simulink model "SchematD"  (Simulink 9.2)
settings: Solver=VariableStepAuto  StartTime=0.0  StopTime=10.0  RelTol=1e-3
libraries: simulink_extras x2
settings Model: Creator=bartl  LastModifiedBy=bartl
settings DataIOCC: LimitDataPoints=off  SaveFormat=Dataset  SignalLoggingSaveFormat=Dataset
settings OptimizationCC: LifeSpan=auto
settings DebuggingCC: UnderspecifiedInitializationDetection=Simplified  MergeDetectMultiDrivingBlocksExec=error  FcnCallInpInsideContextMsg=error  StateNameClashWarn=none  SFUnexpectedBacktrackingDiag=error  SFNoUnconditionalDefaultTransitionDiag=error  SFExecutionAtInitializationDiag=warning
settings HardwareCC: ProdBitPerPointer=64  ProdBitPerSizeT=64  ProdBitPerPtrDiffT=64  ProdLargestAtomicFloat=Float  ProdIntDivRoundTo=Zero  ProdEndianess=LittleEndian  ProdWordSize=64  ProdHWDeviceType=Intel->x86-64 (Windows64)
settings ModelReferenceCC: PropagateSignalLabelsOutOfModel=on
settings SFSimCC: SimUseLocalCustomCode=on
settings RTWCC: RTWUseLocalCustomCode=on
settings CodeAppCC: StateflowObjectComments=off
settings GRTTargetCC: TargetLangStandard=C99 (ISO)  GeneratePreprocessorConditionals=Use local settings  CombineOutputUpdateFcns=on  GRTInterface=off
settings ConfigComp: CovMetricSettings=dwe  CovHtmlReporting=off  CovSaveCumulativeToWorkspaceVar=off  CovSaveSingleToWorkspaceVar=off  CovExternalEMLEnable=on

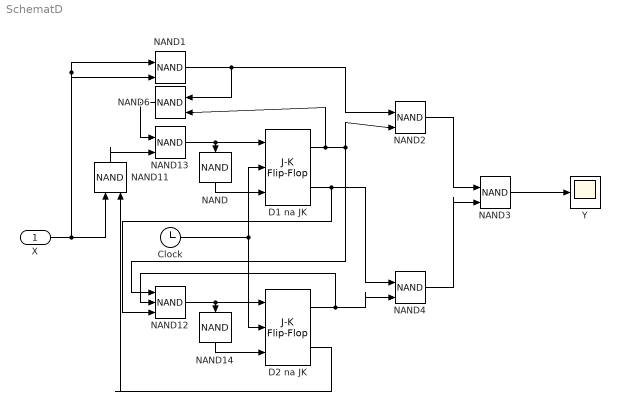
== system SchematD ==
  X : Inport
  Clock : Clock
  D1 na JK : simulink_extras/Flip Flops/J-K Flip-Flop  initial_condition=0
      settings: SourceProductName=Simulink
  D2 na JK : simulink_extras/Flip Flops/J-K Flip-Flop  initial_condition=0
      settings: SourceProductName=Simulink
  NAND : Logic  Operator=NAND  Inputs=1  IconShape=distinctive  AllPortsSameDT=off  OutDataTypeStr=boolean
  NAND{1..4,6,11,13} (7 alike) : Logic  Operator=NAND  IconShape=distinctive  AllPortsSameDT=off  OutDataTypeStr=boolean
  NAND12 : Logic  Operator=NAND  Inputs=3  IconShape=distinctive  AllPortsSameDT=off  OutDataTypeStr=boolean
  NAND14 : Logic  Operator=NAND  Inputs=1  IconShape=distinctive  AllPortsSameDT=off  OutDataTypeStr=boolean
  Y : Scope
  wires:
  NAND/1 -> D1 na JK/3
  NAND14/1 -> D2 na JK/3
  NAND13/1 -> NAND/1, D1 na JK/1
  NAND12/1 -> NAND14/1, D2 na JK/1
  Clock/1 -> D2 na JK/2, D1 na JK/2
  X/1 -> NAND11/1, NAND1/2, NAND1/1
  D1 na JK/1 -> NAND6/2, NAND12/1, NAND2/2
  NAND1/1 -> NAND6/1, NAND2/1
  D2 na JK/1 -> NAND12/2, NAND4/2
  D1 na JK/2 -> NAND12/3, NAND4/1
  NAND2/1 -> NAND3/1
  NAND4/1 -> NAND3/2
  NAND3/1 -> Y/1
  NAND6/1 -> NAND13/1
  NAND11/1 -> NAND13/2
  D2 na JK/2 -> NAND11/2
